simulink model "Heat_pump_Rohan"  (R2023b)
settings: Solver=VariableStepAuto  StartTime=0.0  StopTime=3600*24*365  RelTol=1e-3
values from neighbouring files (symbols this model uses):
  sample_time = 3600    [PV_code.m]    (also in Prof_UAEScode.m; UAES_ws_HP.mat; UAES_ws_PV.mat)
  T_Ambient_dC = 15    [Prof_UAEScode.m]    (also in UAES_ws_HP.mat)
  T_OFF_Heater_dC = 80    [Prof_UAEScode.m]    (also in UAES_ws_HP.mat)
  T_OFF_Room_dC = 19.8    [Prof_UAEScode.m]    (also in UAES_ws_HP.mat)
  T_ON_Heater_dC = 50    [Prof_UAEScode.m]    (also in UAES_ws_HP.mat)
  T_ON_Room_dC = 20.2    [Prof_UAEScode.m]    (also in UAES_ws_HP.mat)
undefined symbols (not defined in the file or in its folder): path_carnot
libraries: carnot x19, simulink x2
settings Model: Creator=Rohan  LastModifiedBy=Rohan

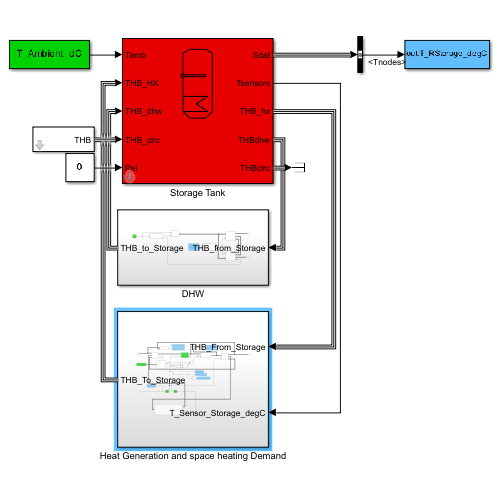
[thumbnail: Simulink's stored preview of the top-level diagram]
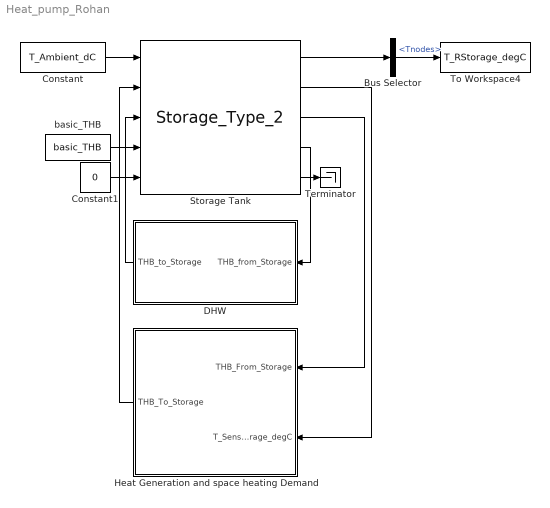
== system Heat_pump_Rohan ==
  Bus Selector : BusSelector  OutputSignals=Tnodes
  Constant : Constant  Value=T_Ambient_dC
  Constant1 : Constant  Value=0
  DHW : Subsystem
  Heat Generation and space heating Demand : Subsystem
  Storage Tank : carnot/Storage/Thermal/Storage_Type_2  t0=[10:5:55]  hgt=1.5719  stgtype=2  tini=[10 15 20 25 30 35 40 45 50 55]  mpts=[1 2 3 4 5 6 7 8 9 10]  PathName=fullfile(path_carnot('libsl'), 'Storage', 'Thermal', 'Storage_Type_2', 'parameter_set')  FileName='<user defined>'  userPath=off  userParam=on  uwall=alpha_Storage_Wm2K  ubot=alpha_Storage_Wm2K  utop=alpha_Storage_Wm2K  axcond=0.5  volume=volume_Storage_m3  dia=diameter_Storage_m  standing=standing cylinder  Tsensor=0.5  nodes=10  mpoints=10  elimthermocline=2  condinvtc=50000  hx1inlet=h_DHW_INLET  hx1outlet=h_HX_OUTLET  hx1dia=d_HX_m  hx1uac=lambda_Storage_WmK  hx1uam=0.15  hx1uat=0.6  uat2=0  hx1dpqua=20  hx1dplin=20  pipe1inlet=h_DHW_INLET  pipe1outlet=h_DHW_OUTLET  pipe1dia=d_DHW_m  pipe2inlet=0.6  pipe2outlet=1  pipe2dia=0.03  heater1start=0  heater1end=0
  Terminator : Terminator
  To Workspace4 : ToWorkspace  VariableName=T_RStorage_degC  SampleTime=sample_time
  basic_THB : carnot/Basic/Hydraulics/basic_THB  t=20  mdot=0  p=1e5  ID=Pressure Drop from Massflow  fluid=Water  mix=0  mix2=0  mix3=0  dia=0.02  hgt=0
  wires:
  Storage Tank/5 -> Terminator/1
  basic_THB/1 -> Storage Tank/4
  Storage Tank/4 -> DHW/1(THB_from_Storage)
  Heat Generation and space heating Demand/1(THB_To_Storage) -> Storage Tank/2
  Storage Tank/1 -> Bus Selector/1
  DHW/1(THB_to_Storage) -> Storage Tank/3
  Constant/1 -> Storage Tank/1
  Storage Tank/3 -> Heat Generation and space heating Demand/1(THB_From_Storage)
  Bus Selector/1 -> To Workspace4/1  "<Tnodes>"
  Constant1/1 -> Storage Tank/5
  Storage Tank/2 -> Heat Generation and space heating Demand/2(T_Sensor_Storage_degC)

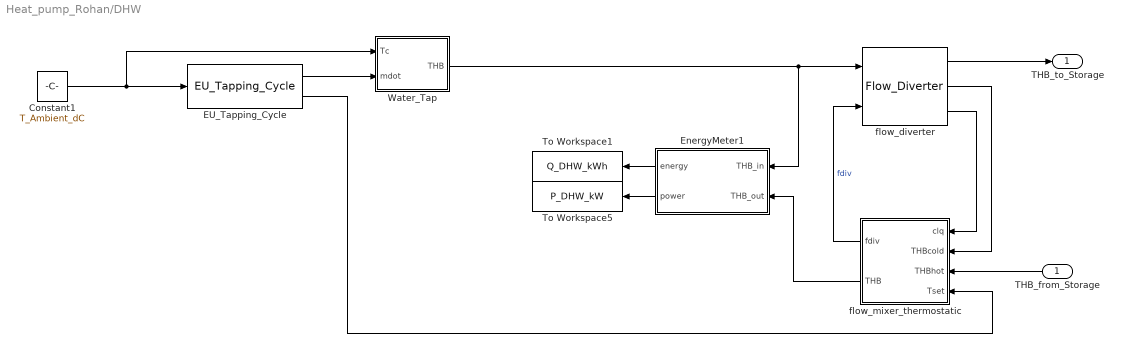
== system Heat_pump_Rohan/DHW ==
  THB_from_Storage : Inport
  Constant1 : Constant  Value=T_Ambient_dC
  EU_Tapping_Cycle : carnot/Load/Hot_Water_Tapping/EU_Tapping_Cycle  eu_tap=M  dTbias=0
  EnergyMeter1 : Subsystem  AncestorBlock=carnot/Control/EnergyMeter  mask(energy meter){}
      mask help: Calculates the power and energy of a fluid flow between inlet and outlet of components.
      mask Help: web(fullfile(path_carnot('help'),'EnergyMeter.html'),'-helpbrowser')
  To Workspace1 : ToWorkspace  VariableName=Q_DHW_kWh  SampleTime=sample_time
  To Workspace5 : ToWorkspace  VariableName=P_DHW_kW  SampleTime=sample_time
  Water_Tap : Subsystem  AncestorBlock=carnot/Load/Hot_Water_Tapping/Water_Tap  mask(water tap){dia=0.02, p=2e5}
      mask prompts: dia "diameter at outlet [m]"; p "system pressure [Pa]"
      mask help:
      | The block models a tap, that produces a constant massflow of a fluid at given times.
      | control = 1 is full massflow, control = 0 is no massflow.
      mask init:
      | fluid = 1; %water
      | mix = 0;
      | dia = max(0.001, dia);
      | p = max(p, 0);
      mask Help: eval('man (''water_tap'')')
      mask Display: plot(-10,10,90,90,[44,67,67,45,45,40,40,44],[80,80,72,72,60,60,76,80],[60,45],[90,90],[53,53],[80,90],[24,29,70,75,24],[30,10,10,30,30],[42,42],[32,58],[46,44],[34,54],[38,40],[34,56])
  flow_diverter : carnot/Hydraulics/Flow_Diverter
  flow_mixer_thermostatic : Subsystem  AncestorBlock=carnot/Hydraulics/Flow_Mixer_Thermostatic  mask(thermostatic flow mixer){t=1}
      mask prompts: t "time constant for valve [s]"
      mask help:
      | The thermostatic flow mixer mixes cold and hot fluid to set a desired temperature and calculates the pressure drop.
      | Use together with flow_diverter_fixed_rate.
      mask init:
      | if t < 0.01
      |     t = 0.01;
      |     disp('Flow mixer thermostatic: time constant set to minimum value 0.01')
      | end
      | t1 = 1/t;
      mask Help: web(fullfile(path_carnot('help'),'Flow_Mixer.html'),'-helpbrowser')
      mask Display: plot(10,0,100,100,[40,60,60,40,40],[60,40,60,40,60],[44,50,56,44],[66,50,66,66],[50,50],[30,50],[56,44],[25,25],[50,50],[10,25])
  THB_to_Storage : Outport
  wires:
  EnergyMeter1/1(energy) -> To Workspace1/1
  flow_diverter/3 -> flow_mixer_thermostatic/1(clq)
  flow_mixer_thermostatic/2(THB) -> EnergyMeter1/2(THB_out)
  EnergyMeter1/2(power) -> To Workspace5/1
  flow_mixer_thermostatic/1(fdiv) -> flow_diverter/2  "fdiv"
  EU_Tapping_Cycle/1 -> Water_Tap/2(mdot)
  Constant1/1 -> Water_Tap/1(Tc), EU_Tapping_Cycle/1
  flow_diverter/2 -> flow_mixer_thermostatic/2(THBcold)
  Water_Tap/1(THB) -> EnergyMeter1/1(THB_in), flow_diverter/1
  EU_Tapping_Cycle/2 -> flow_mixer_thermostatic/4(Tset)
  THB_from_Storage/1 -> flow_mixer_thermostatic/3(THBhot)
  flow_diverter/1 -> THB_to_Storage/1

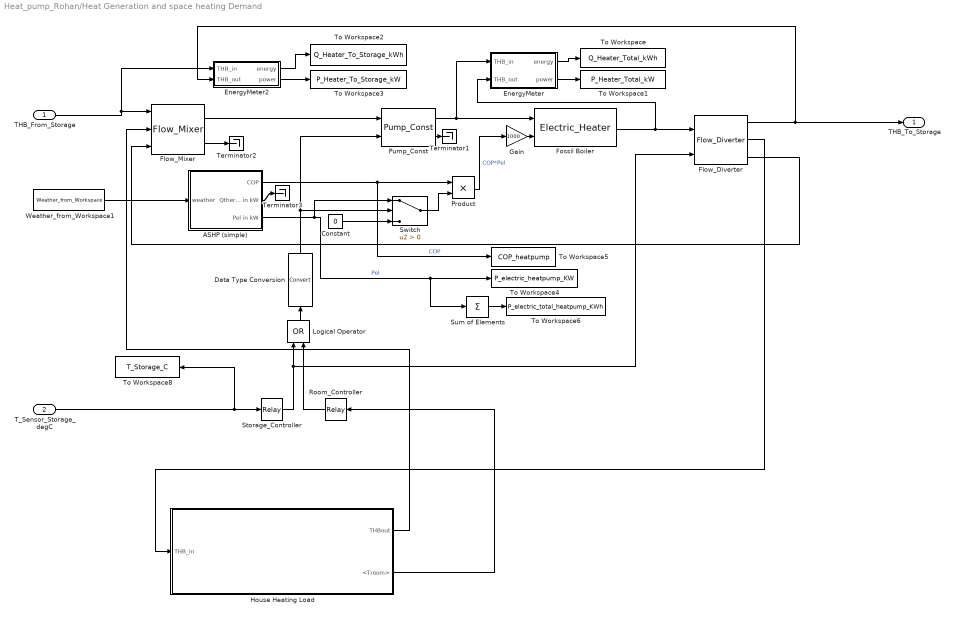
== system Heat_pump_Rohan/Heat Generation and space heating Demand ==
  THB_From_Storage : Inport
  T_Sensor_Storage_degC : Inport  Port=2
  ASHP (simple) : Subsystem
  Constant : Constant  Value=0
  Data Type Conversion : DataTypeConversion  SaturateOnIntegerOverflow=off  RndMeth=Floor
  EnergyMeter : Subsystem  AncestorBlock=carnot/Control/EnergyMeter  mask(energy meter){}
      mask help: Calculates the power and energy of a fluid flow between inlet and outlet of components.
      mask Help: web(fullfile(path_carnot('help'),'EnergyMeter.html'),'-helpbrowser')
  EnergyMeter2 : Subsystem  AncestorBlock=carnot/Control/EnergyMeter  mask(energy meter){}
      mask help: Calculates the power and energy of a fluid flow between inlet and outlet of components.
      mask Help: web(fullfile(path_carnot('help'),'EnergyMeter.html'),'-helpbrowser')
  Flow_Diverter : carnot/Hydraulics/Flow_Diverter
  Flow_Mixer : carnot/Hydraulics/Flow_Mixer  InitialCondition=0.5  TransferFnMode=off  t_fdiv=10
  Fossil Boiler : carnot/Source/Boiler/Electric_Heater
  Gain : Gain  Gain=1000
  House Heating Load : Subsystem
  Logical Operator : Logic  Operator=OR  AllPortsSameDT=off  OutDataTypeStr=boolean
  Product : Product
  Pump_Const : carnot/Hydraulics/Pump_Const  mdotmax=mdot_BCK_kgs  dia=0.02  p0=3e5  fluid_id=Water  mix=0  mix2=0  mix3=0  UA=3  mcp=4182  Tini=20  UpperLimit=1  LowerLimit=0  e0=10  e1=10  e2=-1
  Room_Controller : Relay  OnSwitchValue=T_ON_Room_dC  OffSwitchValue=T_OFF_Room_dC  OnOutputValue=0  OffOutputValue=1
  Storage_Controller : Relay  OnSwitchValue=T_OFF_Heater_dC  OffSwitchValue=T_ON_Heater_dC  OnOutputValue=0  OffOutputValue=1
  Sum of Elements : Sum  Inputs=+
  Switch : Switch  Criteria=u2 > Threshold  SaturateOnIntegerOverflow=off  InputSameDT=off
  Terminator1 : Terminator
  Terminator2 : Terminator
  Terminator3 : Terminator
  To Workspace : ToWorkspace  VariableName=Q_Heater_Total_kWh  SampleTime=sample_time
  To Workspace1 : ToWorkspace  VariableName=P_Heater_Total_kW  SampleTime=sample_time
  To Workspace2 : ToWorkspace  VariableName=Q_Heater_To_Storage_kWh  SampleTime=sample_time
  To Workspace3 : ToWorkspace  VariableName=P_Heater_To_Storage_kW  SampleTime=sample_time
  To Workspace4 : ToWorkspace  VariableName=P_electric_heatpump_KW  SampleTime=sample_time
  To Workspace5 : ToWorkspace  VariableName=COP_heatpump  SampleTime=sample_time
  To Workspace6 : ToWorkspace  VariableName=P_electric_total_heatpump_KWh  SampleTime=sample_time
  To Workspace8 : ToWorkspace  VariableName=T_Storage_C  SampleTime=sample_time
  Weather_from_Workspace1 : carnot/Weather/Weather_from_Workspace  file=weather
  THB_To_Storage : Outport
  wires:
  Logical Operator/1 -> Data Type Conversion/1
  Room_Controller/1 -> Logical Operator/2
  THB_From_Storage/1 -> Flow_Mixer/1, EnergyMeter2/1(THB_in)
  Flow_Diverter/3 -> Flow_Mixer/3
  Data Type Conversion/1 -> Switch/2, Pump_Const/2
  Flow_Mixer/1 -> Pump_Const/1
  Storage_Controller/1 -> Logical Operator/1, Flow_Diverter/2
  Pump_Const/1 -> Fossil Boiler/1, EnergyMeter/1(THB_in)
  Switch/1 -> Product/2
  Flow_Diverter/1 -> THB_To_Storage/1, EnergyMeter2/2(THB_out)
  T_Sensor_Storage_degC/1 -> To Workspace8/1, Storage_Controller/1
  EnergyMeter/1(energy) -> To Workspace/1
  EnergyMeter/2(power) -> To Workspace1/1
  EnergyMeter2/2(power) -> To Workspace3/1
  EnergyMeter2/1(energy) -> To Workspace2/1
  Flow_Mixer/2 -> Terminator2/1
  Constant/1 -> Switch/3
  Pump_Const/2 -> Terminator1/1
  ASHP (simple)/1(COP) -> To Workspace5/1, Product/1  "COP"
  Fossil Boiler/1 -> EnergyMeter/2(THB_out), Flow_Diverter/1
  ASHP (simple)/3(Pel in kW) -> Sum of Elements/1, To Workspace4/1, Switch/1  "Pel"
  Weather_from_Workspace1/1 -> ASHP (simple)/1(weather)
  Product/1 -> Gain/1  "COP*Pel"
  ASHP (simple)/2(Qtherm in kW) -> Terminator3/1
  Gain/1 -> Fossil Boiler/2
  Flow_Diverter/2 -> House Heating Load/1(THB_in)
  House Heating Load/1(THBout) -> Flow_Mixer/2
  House Heating Load/2(<Troom>) -> Room_Controller/1
  Sum of Elements/1 -> To Workspace6/1

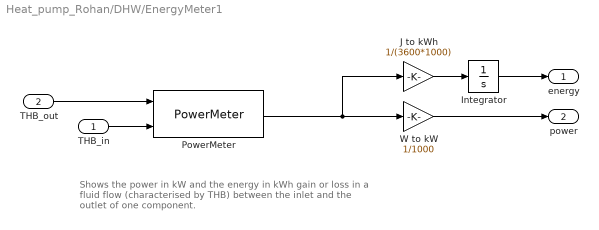
== system Heat_pump_Rohan/DHW/EnergyMeter1 ==
  note: Shows the power in kW and the energy in kWh gain or loss
      | in a fluid flow (characterised by THB) between the
      | inlet and the outlet of one component.
  THB_in : Inport
  THB_out : Inport  Port=2
  Integrator : Integrator  UpperSaturationLimit=1  LowerSaturationLimit=0
  J to kWh : Gain  Gain=1/(3600*1000)
  PowerMeter : carnot/Control/PowerMeter
  W to kW : Gain  Gain=1/1000
  energy : Outport
  power : Outport  Port=2
  wires:
  PowerMeter/1 -> W to kW/1, J to kWh/1
  THB_in/1 -> PowerMeter/2
  Integrator/1 -> energy/1
  THB_out/1 -> PowerMeter/1
  J to kWh/1 -> Integrator/1
  W to kW/1 -> power/1

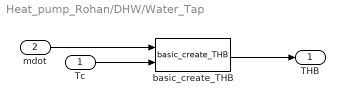
== system Heat_pump_Rohan/DHW/Water_Tap ==
  Tc : Inport
  mdot : Inport  Port=2
  basic_create_THB : carnot/Basic/Hydraulics/basic_create_THB  p=p  fluid=Water  mix=mix  mix2=0  mix3=0  dia=dia  hgt=0  mID=No Pressure Drop
  THB : Outport
  wires:
  basic_create_THB/1 -> THB/1
  Tc/1 -> basic_create_THB/2
  mdot/1 -> basic_create_THB/1

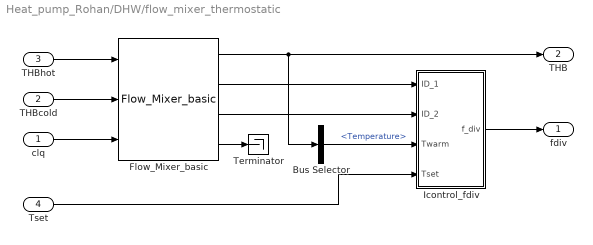
== system Heat_pump_Rohan/DHW/flow_mixer_thermostatic ==
  clq : Inport
  THBcold : Inport  Port=2
  THBhot : Inport  Port=3
  Tset : Inport  Port=4
  Bus Selector : BusSelector  OutputSignals=Temperature
  Flow_Mixer_basic : carnot/Basic/Hydraulics/Flow_Mixer_basic
  Icontrol_fdiv : Subsystem
  Terminator : Terminator
  fdiv : Outport
  THB : Outport  Port=2
  wires:
  Icontrol_fdiv/1(f_div) -> fdiv/1
  THBhot/1 -> Flow_Mixer_basic/1
  THBcold/1 -> Flow_Mixer_basic/2
  clq/1 -> Flow_Mixer_basic/3
  Flow_Mixer_basic/1 -> THB/1, Bus Selector/1
  Flow_Mixer_basic/2 -> Icontrol_fdiv/1(ID_1)
  Flow_Mixer_basic/3 -> Icontrol_fdiv/2(ID_2)
  Tset/1 -> Icontrol_fdiv/4(Tset)
  Flow_Mixer_basic/4 -> Terminator/1
  Bus Selector/1 -> Icontrol_fdiv/3(Twarm)  "<Temperature>"

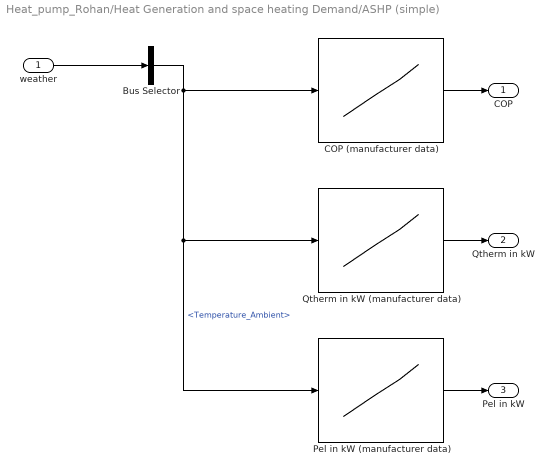
== system Heat_pump_Rohan/Heat Generation and space heating Demand/ASHP (simple) ==
  weather : Inport
  Bus Selector : BusSelector  OutputSignals=Temperature_Ambient
  COP (manufacturer data) : Lookup_n-D  NumberOfTableDimensions=1  BreakpointsForDimension1=[-15 -10 -7 -2 2 7 12 15 20 25 27 31 35 ]  BreakpointsForDimension2=|  Table=[1.28,1.61,1.82,2.09,2.29,2.85,3.04,3.30,3.77,4.24,4.43,4.80,5.18]  InternalRulePriority=Speed  RndMeth=Simplest
      | [40 45 50 55
      | 55 55 55 55 55 60 60 ]
  Pel in kW (manufacturer data) : Lookup_n-D  NumberOfTableDimensions=1  BreakpointsForDimension1=[-15 -10 -7 -2 2 7 12 15 20 23 27 31]  BreakpointsForDimension2=|  Table=[2.4 2.4 2.4 2.2 2.0 1.8 1.5 1.5 1.5 1 1 1]  InternalRulePriority=Speed  RndMeth=Simplest
      | [30 35 40 45 50 55
      | ]
  Qtherm in kW (manufacturer data) : Lookup_n-D  NumberOfTableDimensions=1  BreakpointsForDimension1=[-15 -10 -7 -2 2 7 12 15 20]  BreakpointsForDimension2=|  Table=[2.6 3.4 3.8 4.1 4.3 4.5 4.6 4.6 4.9]  InternalRulePriority=Speed  RndMeth=Simplest
      | [30 35 40 45 50 55
      | ]
  COP : Outport  VectorParamsAs1DForOutWhenUnconnected=off
  Qtherm in kW : Outport  Port=2  VectorParamsAs1DForOutWhenUnconnected=off
  Pel in kW : Outport  Port=3  VectorParamsAs1DForOutWhenUnconnected=off
  wires:
  weather/1 -> Bus Selector/1
  Qtherm in kW (manufacturer data)/1 -> Qtherm in kW/1
  Pel in kW (manufacturer data)/1 -> Pel in kW/1
  COP (manufacturer data)/1 -> COP/1
  Bus Selector/1 -> Pel in kW (manufacturer data)/1, Qtherm in kW (manufacturer data)/1, COP (manufacturer data)/1  "<Temperature_Ambient>"

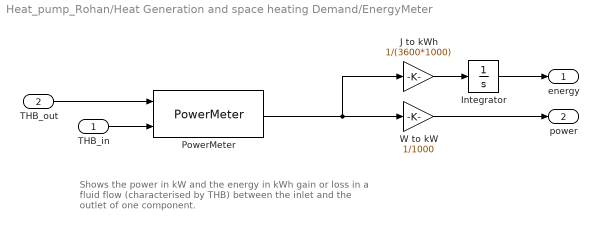
== system Heat_pump_Rohan/Heat Generation and space heating Demand/EnergyMeter ==
  note: Shows the power in kW and the energy in kWh gain or loss
      | in a fluid flow (characterised by THB) between the
      | inlet and the outlet of one component.
  THB_in : Inport
  THB_out : Inport  Port=2
  Integrator : Integrator  UpperSaturationLimit=1  LowerSaturationLimit=0
  J to kWh : Gain  Gain=1/(3600*1000)
  PowerMeter : carnot/Control/PowerMeter
  W to kW : Gain  Gain=1/1000
  energy : Outport
  power : Outport  Port=2
  wires:
  PowerMeter/1 -> W to kW/1, J to kWh/1
  THB_in/1 -> PowerMeter/2
  Integrator/1 -> energy/1
  THB_out/1 -> PowerMeter/1
  J to kWh/1 -> Integrator/1
  W to kW/1 -> power/1

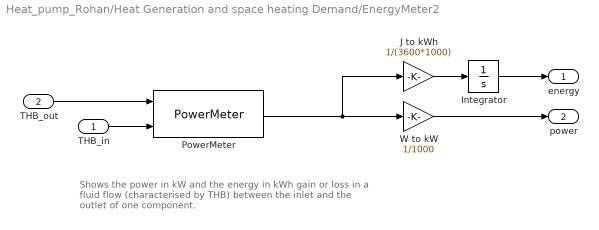
== system Heat_pump_Rohan/Heat Generation and space heating Demand/EnergyMeter2 ==
  note: Shows the power in kW and the energy in kWh gain or loss
      | in a fluid flow (characterised by THB) between the
      | inlet and the outlet of one component.
  THB_in : Inport
  THB_out : Inport  Port=2
  Integrator : Integrator  UpperSaturationLimit=1  LowerSaturationLimit=0
  J to kWh : Gain  Gain=1/(3600*1000)
  PowerMeter : carnot/Control/PowerMeter
  W to kW : Gain  Gain=1/1000
  energy : Outport
  power : Outport  Port=2
  wires:
  PowerMeter/1 -> W to kW/1, J to kWh/1
  THB_in/1 -> PowerMeter/2
  Integrator/1 -> energy/1
  THB_out/1 -> PowerMeter/1
  J to kWh/1 -> Integrator/1
  W to kW/1 -> power/1

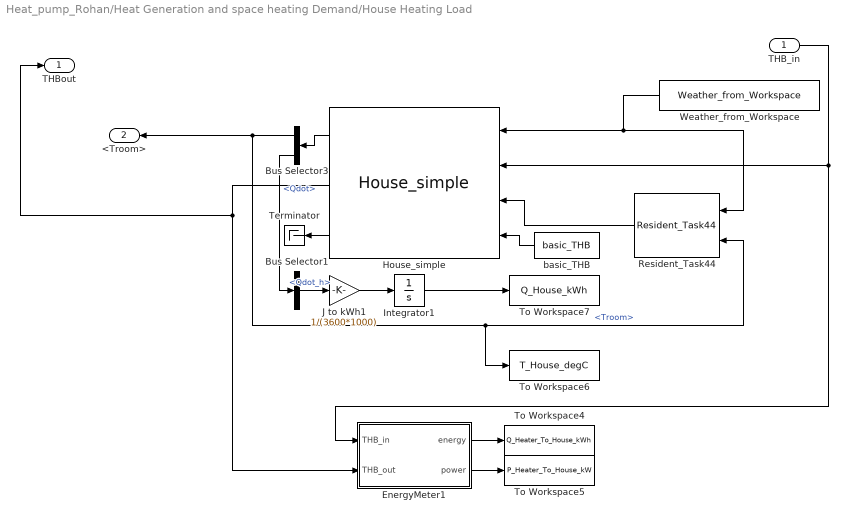
== system Heat_pump_Rohan/Heat Generation and space heating Demand/House Heating Load ==
  THB_in : Inport
  Bus Selector1 : BusSelector  OutputSignals=Qdot_h
  Bus Selector3 : BusSelector  OutputSignals=Troom,Qdot
  EnergyMeter1 : Subsystem  AncestorBlock=carnot/Control/EnergyMeter  mask(energy meter){}
      mask help: Calculates the power and energy of a fluid flow between inlet and outlet of components.
      mask Help: web(fullfile(path_carnot('help'),'EnergyMeter.html'),'-helpbrowser')
  House_simple : carnot/Load/Houses/House_simple  tini=20  CO2init=400  VOCinit=0  calcAir=off  dtroom=inf  Tmeaninside=23.8  deltathetai=3.8  Tmeanoutside=11  deltathetae=9.3  tshift=319*3600  PathName=fullfile(path_carnot('libsl'), 'Load', 'Houses', 'House_simple', 'parameter_set')  FileName='<user defined>'  userPath=off  userParam=on  Ahabit=210  Hroom=2.5  slabwidth=10  slablength=7  dwall=0.4  UAwall=80.775  capa=500000  utot=0.227  gammat=0  cond_ground=2  cp_ground=800  rho_ground=2500  Awindow=[0.36 0.36 0.36 0.36 ]  AziWin=[0 90 -180 -90]  Uwindow=[1.2 1.2 1.2 1.2]  Gwindow=[0.5 0.5 0.5 0.5]  alpha=10  H=0.6  W=0.6  Nwin=4  Ventilationrate=0.4  Heatrecovery=0.8  pnom=10000  dtnom=49.83  expo=1.3  mcap=10*4812  lin=100  qua=100
  Integrator1 : Integrator  UpperSaturationLimit=1  LowerSaturationLimit=0
  J to kWh1 : Gain  Gain=1/(3600*1000)
  Resident_Task44 : carnot/Load/Houses/Resident_Task44  period=24*3600  rep_seq_te=[0 1 6 7 8 9 11 12 13 18 19 20 22 23]*3600  rep_seq_de=[1 5 1 1 1 2 1 1 4 2 1 2 1 1]*3600  rep_seq_ye=[105 55 392.5 457.5 420 55 250 55 120 170 615 420 442.5 355]  rep_seq_to=[0 6 7 8 9 11 12 13 14 15 17 18 20 21 22]*3600  rep_seq_do=[6 1 1 1 2 1 1 1 1 2 1 2 1 1 2]*3600  rep_seq_yo=[4 2 3 2 0 1 3 2 1 0 1 2 4 3 4]*60  rep_seq_yco2="[4 2 3 2 0 1 3 2 1 0 1 2 4 3 4]*0.005/60*0.04  % 5 liter/person/minute with 4 % CO2"  rep_seq_yvoc=[4 2 3 2 0 1 3 2 1 0 1 2 4 3 4]*0.001/3600 % 1 g/person/hour  rep_seq_yh2o=[4 2 3 2 0 1 3 2 1 0 1 2 4 3 4]*0.001/60 % 1 g/person/minute  Topen=30  Tclose=30  TrAboveTa=20  TaTooCold=12  timeFIR=24  TaIni=12  starttime=8  stoptime=22  TroomShadeOn=30  TroomShadeOff=22.8  SolarShadeOn=300  SolarShadeOff=200  max_shade=1
  Terminator : Terminator
  To Workspace4 : ToWorkspace  VariableName=Q_Heater_To_House_kWh  SampleTime=sample_time
  To Workspace5 : ToWorkspace  VariableName=P_Heater_To_House_kW  SampleTime=sample_time
  To Workspace6 : ToWorkspace  VariableName=T_House_degC  SampleTime=sample_time
  To Workspace7 : ToWorkspace  VariableName=Q_House_kWh  SampleTime=sample_time
  Weather_from_Workspace : carnot/Weather/Weather_from_Workspace  file=weather
  basic_THB : carnot/Basic/Hydraulics/basic_THB  t=20  mdot=0  p=1e5  ID=Pressure Drop from Massflow  fluid=Water  mix=0  mix2=0  mix3=0  dia=0.02  hgt=0
  THBout : Outport
  <Troom> : Outport  Port=2
  wires:
  House_simple/1 -> Bus Selector3/1
  House_simple/2 -> THBout/1, EnergyMeter1/2(THB_out)
  basic_THB/1 -> House_simple/4
  Bus Selector1/1 -> J to kWh1/1  "<Qdot_h>"
  Weather_from_Workspace/1 -> Resident_Task44/1, House_simple/1
  Bus Selector3/1 -> <Troom>/1, To Workspace6/1, Resident_Task44/2  "<Troom>"
  Integrator1/1 -> To Workspace7/1
  House_simple/3 -> Terminator/1
  EnergyMeter1/2(power) -> To Workspace5/1
  EnergyMeter1/1(energy) -> To Workspace4/1
  Resident_Task44/1 -> House_simple/3
  Bus Selector3/2 -> Bus Selector1/1  "<Qdot>"
  THB_in/1 -> EnergyMeter1/1(THB_in), House_simple/2
  J to kWh1/1 -> Integrator1/1

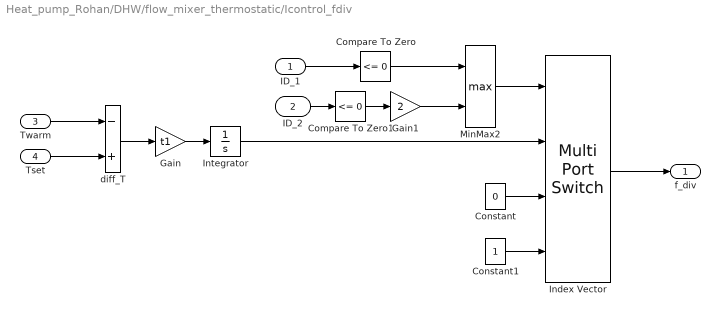
== system Heat_pump_Rohan/DHW/flow_mixer_thermostatic/Icontrol_fdiv ==
  ID_1 : Inport
  ID_2 : Inport  Port=2
  Twarm : Inport  Port=3
  Tset : Inport  Port=4
  Compare To Zero : simulink/Logic and Bit Operations/Compare To Zero  relop=<=  OutDataTypeStr=uint8
  Compare To Zero1 : simulink/Logic and Bit Operations/Compare To Zero  relop=<=  OutDataTypeStr=uint8
  Constant : Constant  Value=0
  Constant1 : Constant
  Gain : Gain  Gain=t1  SaturateOnIntegerOverflow=on  OutDataTypeStr=Inherit: Same as input  ParamDataTypeStr=Inherit: Same as input
  Gain1 : Gain  Gain=2
  Index Vector : MultiPortSwitch  DataPortOrder=Zero-based contiguous  zeroidx=on  SaturateOnIntegerOverflow=off  InputSameDT=off
  Integrator : Integrator  LimitOutput=on  UpperSaturationLimit=1  LowerSaturationLimit=0
  MinMax2 : MinMax  Function=max  Inputs=2
  diff_T : Sum  Inputs=-+  InputSameDT=on  SaturateOnIntegerOverflow=on  OutDataTypeStr=Inherit: Same as first input
  f_div : Outport
  wires:
  Compare To Zero1/1 -> Gain1/1
  Compare To Zero/1 -> MinMax2/1
  MinMax2/1 -> Index Vector/1
  ID_1/1 -> Compare To Zero/1
  ID_2/1 -> Compare To Zero1/1
  Constant/1 -> Index Vector/3
  Integrator/1 -> Index Vector/2
  Constant1/1 -> Index Vector/4
  Gain1/1 -> MinMax2/2
  Index Vector/1 -> f_div/1
  Tset/1 -> diff_T/2
  Twarm/1 -> diff_T/1
  Gain/1 -> Integrator/1
  diff_T/1 -> Gain/1

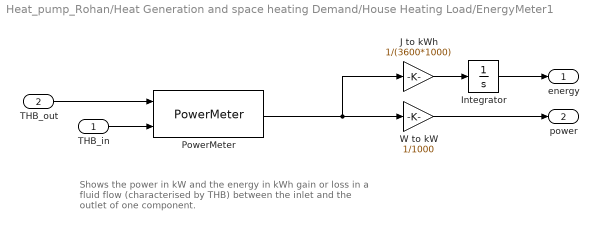
== system Heat_pump_Rohan/Heat Generation and space heating Demand/House Heating Load/EnergyMeter1 ==
  note: Shows the power in kW and the energy in kWh gain or loss
      | in a fluid flow (characterised by THB) between the
      | inlet and the outlet of one component.
  THB_in : Inport
  THB_out : Inport  Port=2
  Integrator : Integrator  UpperSaturationLimit=1  LowerSaturationLimit=0
  J to kWh : Gain  Gain=1/(3600*1000)
  PowerMeter : carnot/Control/PowerMeter
  W to kW : Gain  Gain=1/1000
  energy : Outport
  power : Outport  Port=2
  wires:
  PowerMeter/1 -> W to kW/1, J to kWh/1
  THB_in/1 -> PowerMeter/2
  Integrator/1 -> energy/1
  THB_out/1 -> PowerMeter/1
  J to kWh/1 -> Integrator/1
  W to kW/1 -> power/1
